simulink model "ex4"  (R2015a)
settings: Solver=ode45  StartTime=0.0  StopTime=10.0  RelTol=1e-3
undefined symbols (not defined in the file): g, l
settings Model: Creator=fschalle  LastModifiedBy=fschalle

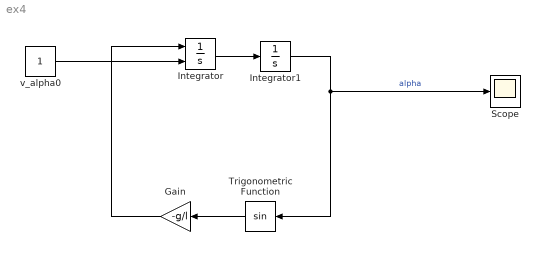
== system ex4 ==
  Gain : Gain  Gain=-g/l
  Integrator : Integrator  InitialConditionSource=external
  Integrator1 : Integrator
  Scope : Scope
  Trigonometric Function : Trigonometry
  "v_alpha0 " : Constant
  wires:
  Integrator/1 -> Integrator1/1
  Integrator1/1 -> Trigonometric Function/1, Scope/1  "alpha"
  "v_alpha0 "/1 -> Integrator/2
  Trigonometric Function/1 -> Gain/1
  Gain/1 -> Integrator/1
